simulink model "KalmanModelSim2"  (R2016b)
settings: Solver=FixedStepAuto  StartTime=0.0  StopTime=t  FixedStep=0.05  RelTol=1e-3
model workspace (MAT data in the model file):
  index = Simulink.Signal
  index.DataType = 'double'
  index.Dimensions = 1
  index.DimensionsMode = 'Fixed'
  index.Complexity = 'real'
  index.SampleTime = -1
  index.SamplingMode = 'auto'
  index.InitialValue = '1'
values from neighbouring files (symbols this model uses):
  dpitch = 7.203    [Parameters.m]
  droll = 0.1094    [Parameters.m]
  dx = 2.86    [Parameters.m]
  dy = 32.5    [Parameters.m]
  dyaw = 0.21285    [Parameters.m]
  Ix = 0.06541    [Parameters.m]
  Iy = 1.08921    [Parameters.m]
  Iz = 1.10675    [Parameters.m]
  l1 = 0.05    [Parameters.m]
  l2 = 0.05    [Parameters.m]
  mx = m    (= 13)    [Parameters.m]
  my = m    (= 13)    [Parameters.m]
  pitch_init = 0    [KF_Position.m]    (also in KalmanModel.m)
  roll_init = 0    [KF_Position.m]    (also in KalmanModel.m)
  Ts = 0.05    [Parameters.m]
  yaw_init = 0    [KF_Position.m]    (also in KalmanModel.m = 0.3)
libraries: simulink x2
settings Model: Creator=USUARIO  LastModifiedBy=USUARIO
settings DataIOCC: Refine=100

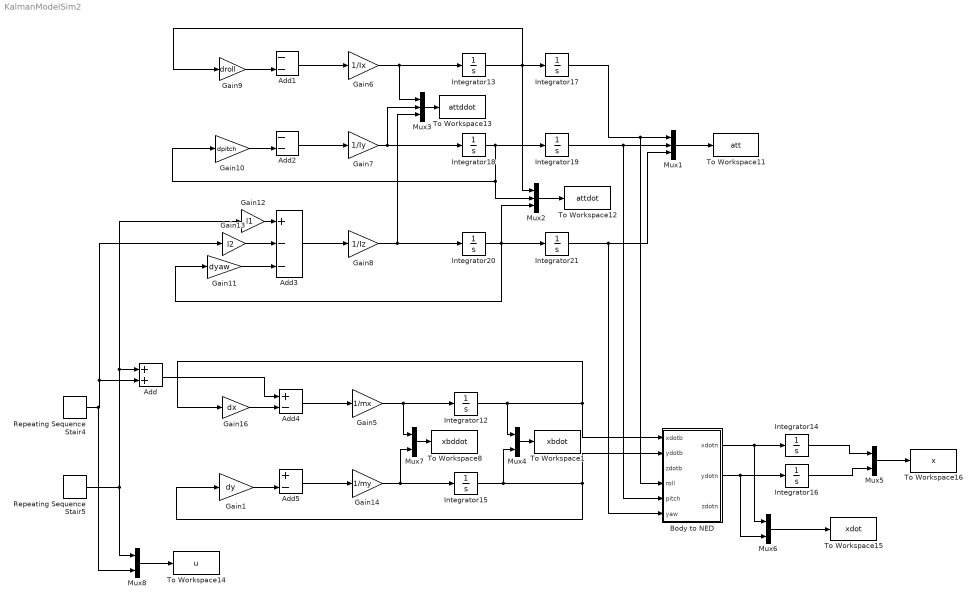
== system KalmanModelSim2 ==
  Add : Sum
  Add1 : Sum  Inputs=--
  Add2 : Sum  Inputs=--
  Add3 : Sum  Inputs=+--
  Add4 : Sum  Inputs=+-
  Add5 : Sum  Inputs=+-
  Body to NED : MATLAB Function  TreatAsAtomicUnit=on
  Gain1 : Gain  Gain=dy
  Gain10 : Gain  Gain=dpitch
  Gain11 : Gain  Gain=dyaw
  Gain12 : Gain  Gain=l1
  Gain13 : Gain  Gain=l2
  Gain14 : Gain  Gain=1/my
  Gain16 : Gain  Gain=dx
  Gain5 : Gain  Gain=1/mx
  Gain6 : Gain  Gain=1/Ix
  Gain7 : Gain  Gain=1/Iy
  Gain8 : Gain  Gain=1/Iz
  Gain9 : Gain  Gain=droll
  Integrator{12..16,18,20} (7 alike) : Integrator
  Integrator17 : Integrator  InitialCondition=roll_init
  Integrator19 : Integrator  InitialCondition=pitch_init
  Integrator21 : Integrator  InitialCondition=yaw_init
  Mux1 : Mux  Inputs=3
  Mux2 : Mux  Inputs=3
  Mux3 : Mux  Inputs=3
  Mux{4..8} (5 alike) : Mux  Inputs=2
  Repeating Sequence Stair4 : simulink/Sources/Repeating Sequence Stair  OutValues=[1 1 0 0].'  tsamp=5  OutMin=[]  OutMax=[]  OutDataTypeStr=double  OutputDataTypeScalingMode=double  OutDataType=fixdt(0,8)  ConRadixGroup=Best Precision: Vector-wise  OutScaling=2^-12
  Repeating Sequence Stair5 : simulink/Sources/Repeating Sequence Stair  OutValues=[0 0 1 1].'  tsamp=5  OutMin=[]  OutMax=[]  OutDataTypeStr=double  OutputDataTypeScalingMode=double  OutDataType=fixdt(0,8)  ConRadixGroup=Best Precision: Vector-wise  OutScaling=2^-12
  To Workspace1 : ToWorkspace  VariableName=xbdot  SaveFormat=Timeseries  SampleTime=Ts
  To Workspace11 : ToWorkspace  VariableName=att  SaveFormat=Timeseries  SampleTime=Ts
  To Workspace12 : ToWorkspace  VariableName=attdot  SaveFormat=Timeseries  SampleTime=Ts
  To Workspace13 : ToWorkspace  VariableName=attddot  SaveFormat=Timeseries  SampleTime=Ts
  To Workspace14 : ToWorkspace  VariableName=u  SaveFormat=Timeseries  SampleTime=Ts
  To Workspace15 : ToWorkspace  VariableName=xdot  SaveFormat=Timeseries  SampleTime=Ts
  To Workspace16 : ToWorkspace  VariableName=x  SaveFormat=Timeseries  SampleTime=Ts
  To Workspace8 : ToWorkspace  VariableName=xbddot  SaveFormat=Timeseries  SampleTime=Ts
  wires:
  Gain6/1 -> Integrator13/1, Mux3/1
  Gain7/1 -> Integrator18/1, Mux3/2
  Gain8/1 -> Mux3/3, Integrator20/1
  Integrator19/1 -> Mux1/2, Body to NED/5(pitch)
  Integrator17/1 -> Mux1/1, Body to NED/4(roll)
  Integrator21/1 -> Body to NED/6(yaw), Mux1/3
  Mux1/1 -> To Workspace11/1
  Mux2/1 -> To Workspace12/1
  Mux3/1 -> To Workspace13/1
  Integrator13/1 -> Gain9/1, Integrator17/1, Mux2/1
  Integrator18/1 -> Mux2/2, Gain10/1, Integrator19/1
  Add1/1 -> Gain6/1
  Add2/1 -> Gain7/1
  Gain10/1 -> Add2/2
  Gain12/1 -> Add3/1
  Add3/1 -> Gain8/1
  Gain11/1 -> Add3/3
  Gain13/1 -> Add3/2
  Gain9/1 -> Add1/2
  Integrator20/1 -> Mux2/3, Integrator21/1, Gain11/1
  Gain5/1 -> Integrator12/1, Mux7/1
  Gain14/1 -> Integrator15/1, Mux7/2
  Integrator16/1 -> Mux5/2
  Integrator14/1 -> Mux5/1
  Mux5/1 -> To Workspace16/1
  Mux6/1 -> To Workspace15/1
  Mux7/1 -> To Workspace8/1
  Add4/1 -> Gain5/1
  Add5/1 -> Gain14/1
  Gain1/1 -> Add5/2
  Gain16/1 -> Add4/2
  Mux8/1 -> To Workspace14/1
  Body to NED/1(xdotn) -> Mux6/1, Integrator14/1
  Body to NED/2(ydotn) -> Mux6/2, Integrator16/1
  Add/1 -> Add4/1
  Repeating Sequence Stair5/1 -> Mux8/1, Gain12/1, Add/1
  Repeating Sequence Stair4/1 -> Mux8/2, Add/2, Gain13/1
  Integrator12/1 -> Mux4/1, Gain16/1, Body to NED/1(xdotb)
  Integrator15/1 -> Body to NED/2(ydotb), Gain1/1, Mux4/2
  Mux4/1 -> To Workspace1/1

== matlab function KalmanModelSim2/Body to NED ==
  data: xdotb input; xdotn output; ydotb input; zdotb input; roll input; pitch input; yaw input; ydotn output; zdotn output
function [xdotn,ydotn,zdotn] = fcn(xdotb,ydotb,zdotb,roll,pitch,yaw)
R=[cos(pitch)*cos(yaw) sin(roll)*sin(pitch)*cos(yaw)-cos(roll)*sin(yaw) ...
                          cos(roll)*sin(pitch)*cos(yaw)+sin(roll)*sin(yaw);
   cos(pitch)*sin(yaw) sin(roll)*sin(pitch)*sin(yaw)+cos(roll)*cos(yaw) ...
                          cos(roll)*sin(pitch)*sin(yaw)-sin(roll)*cos(yaw);
   -sin(pitch) sin(roll)*cos(pitch) cos(roll)*cos(pitch)];

n=R*[xdotb;ydotb;zdotb];

xdotn=n(1);
ydotn=n(2);
zdotn=n(3);
end
